simulink model "doc_convcoding"  (Simulink 6.0)
settings: Solver=ode45  StartTime=0.0  StopTime=inf  RelTol=1e-3
undefined symbols (not defined in the file): slcm
libraries: commcnvcod2 x2, commrandsrc2 x1, commchan2 x1, commsink2 x1
settings Model: Creator=skeene  LastModifiedBy=agaltman  BlockReductionOpt=off  ZeroCrossControl=UseLocalSettings  ProdHWDeviceType=Microprocessor  TargetHWChar=2  TargetHWWordLengths=8,16,32,32  RTWMathFcnLibMatFile=iso_c_tmw.mat  RTWOptions="-aEnforceIntegerDowncast=1 -aFoldNonRolledExpr=1 -aInlineInvariantSignals=1 -aInlineParameters=0 -aLocalBlockOutputs=1 -aRollThreshold=5 -aGenerateReport=0 -aGenCodeOnly=0 -aRTWVerbose=1 -aForceParamTrailComments=0 -aGenerateComments=1 -aIgnoreCustomStorageClasses=1 -aIncHierarchyInIds=0 -aMaxRTWIdLen=31 -aShowEliminatedStatements=0 -aPrefixModelToSubsysFcnNames=1 -aIncDataTypeInIds=0 -aInlinedPrmAccess=\"Literals\" -aTargetFcnLib=\"iso_c_tmw.mat\" -aGenerateFullHeader=1 -aIsPILTarget=0 -aExtMode=0 -aExtModeStaticAlloc=0 -aExtModeTesting=0 -aExtModeStaticAllocSize=1000000 -aExtModeTransport=0 -aLogVarNameModifier=\"rt_\" -aRTWCAPISignals=0 -aRTWCAPIParams=0"
settings DataIOCC: SignalLoggingName=sigsOut
settings OptimizationCC: BlockReduction=off  BooleanDataType=off  MultiInstanced=off
settings FormatCC: IgnoreBidirectionalLines=off
settings HardwareCC: ProdHWDeviceType=Microprocessor  ShiftRightIntArith=on  TargetHWCharacteristics=InheritFromRTWHook
settings CodeAppCC: FileBanners=off
settings GRTTargetCC: TargetFcnLib=iso_c_tmw.mat  IsERTTarget=off

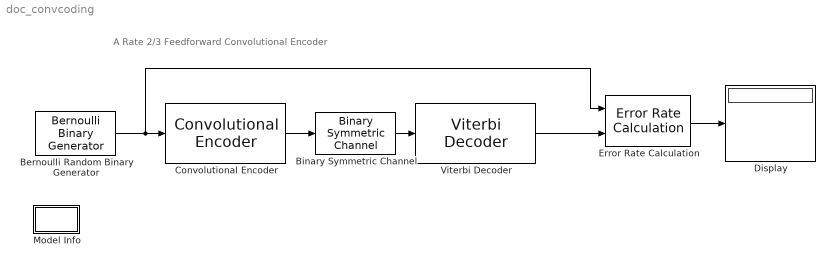
== system doc_convcoding ==
  note: A Rate 2/3 Feedforward Convolutional Encoder
  Bernoulli Random Binary Generator : commrandsrc2/Bernoulli Binary Generator  P=.5  seed=129499  Ts=.5  frameBased=on  sampPerFrame=2  orient=off
  Binary Symmetric Channel : commchan2/Binary Symmetric Channel  P=0.02  s=149  E=off
  Convolutional Encoder : commcnvcod2/Convolutional Encoder  trellis=poly2trellis([5 4], [23 35 0; 0 5 13] )  reset=None
  Display : Display
  Error Rate Calculation : commsink2/Error Rate Calculation  N=68  st_delay=0  cp_mode=Entire frame  subframe=[]  PMode=Port  WsName=ErrorVec  RsMode2=off  stop=on  numErr=100  maxBits=1e6
  Model Info : Subsystem  LoadFcn=slcm LoadBlock;  InitFcn=slcm('UpdateAllCMBlocksInThisModelInit')  mask(CMBlock){InitialSaveTempField=, InitialBlockCM=none, BlockCM=none, Frame=on, SaveTempField=, DisplayStringWithTags=Info, MaskDisplayString=Info, HorizontalTextAlignment=Center, LeftAlignmentValue=0.5, SourceBlockDiagram=doc_convcoding, TagMaxNumber=20, CMTag1=, CMTag2=, CMTag3=, CMTag4=, CMTag5=, CMTag6=, CMTag7=, CMTag8=, CMTag9=, CMTag10=, CMTag11=, CMTag12=, CMTag13=, CMTag14=, CMTag15=, CMTag16=, CMTag17=, CMTag18=, CMTag19=, CMTag20=}
      mask help: This block allows revision control information to be displayed within the model.
      settings: CopyFcn=slcm CopyBlock;  DeleteFcn=slcm Cancel;  PostSaveFcn=slcm('UpdateAllCMBlocksInThisModel')  NameChangeFcn=slcm Rename;  OpenFcn=commdemohelp;
      mask Display: text(str2num(LeftAlignmentValue), 0.5, MaskDisplayString, 'HorizontalAlignment', HorizontalTextAlignment)
  Viterbi Decoder : commcnvcod2/Viterbi Decoder  trellis=poly2trellis([5 4], [23 35 0; 0 5 13] )  dectype=Hard Decision  nsdecb=4  tbdepth=34  opmode=Continuous  reset=off
  wires:
  Convolutional Encoder/1 -> Binary Symmetric Channel/1
  Binary Symmetric Channel/1 -> Viterbi Decoder/1
  Error Rate Calculation/1 -> Display/1
  Bernoulli Random Binary Generator/1 -> Convolutional Encoder/1, Error Rate Calculation/1
  Viterbi Decoder/1 -> Error Rate Calculation/2

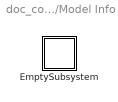
== system doc_convcoding/Model Info ==
  EmptySubsystem : Subsystem

== system doc_convcoding/Model Info/EmptySubsystem ==
